simulink model "Observer_design"  (R2022a)
settings: Solver=ode45  StartTime=0.0  StopTime=30  RelTol=1e-3
values from neighbouring files (symbols this model uses):
  A = [0 0 1 0 0 ... (first row only)    [DesignProjectP2.m]    (also in DesignProjectP3.m; DesignProject_OffsetP3.m; mpc_example_regulation.m = [ 	 0,       0,              1,  0, 0; 	 0,       0,        ; mpc_example_tracking.m = [ 	 0,       0,              1,  0, 0; 	 0,       0,        )
  A_11 = A_measured(:,1:2)    [DesignProjectP2.m]
  A_12 = A_measured(:,3:5)    [DesignProjectP2.m]
  A_21 = A_estimated(:,1:2)    [DesignProjectP2.m]
  A_22 = A_estimated(:,3:5)    [DesignProjectP2.m]
  absolute_encoder_counts_per_revolution = 4096    [ELEN90064_Project_Parameters.m]
  B = [0;0;0;0;1/La]    [DesignProjectP2.m]    (also in DesignProjectP3.m; DesignProject_OffsetP3.m; mpc_example_regulation.m = [0; 0; 0; 0; 1/La]; mpc_example_tracking.m = [0; 0; 0; 0; 1/La])
  B_1 = [Dp.b(1); Dp.b(2)]    [DesignProjectP2.m]
  B_2 = [Dp.b(3); Dp.b(4); Dp.b(5)]    [DesignProjectP2.m]
  C = [1 0 0 0 0 ... (first row only)    [DesignProjectP2.m]    (also in DesignProjectP3.m; DesignProject_OffsetP3.m; mpc_example_regulation.m; mpc_example_tracking.m)
  Dp = c2d(Gp, T, 'zoh')    [DesignProjectP2.m]    (also in DesignProject_OffsetP3.m; mpc_example_regulation.m; mpc_example_tracking.m)
  init = [theta_m_init; theta_l_init; thetadot_m_init; thetadot_l_init; Ia_init]    [ELEN90064_Project_Parameters.m]
  J_r = place(A_22', A_12', obsz)'    [DesignProjectP2.m]
  L = place(A', C', observer_poles)'    [DesignProjectP2.m]    (also in DesignProjectP3.m; DesignProject_OffsetP3.m = L_t'; phase2_emc.m = place(A',C',desired_obsv_poles)')
  T = 1/50    (= 0.02)    [DesignProjectP2.m]    (also in DesignProject_OffsetP3.m; mpc_example_regulation.m; mpc_example_tracking.m)
  theta_l_init = deg2rad(0)    [ELEN90064_Project_Parameters.m]    (also in mpc_example_regulation.m; mpc_example_tracking.m)
  vision_fps = 50    [ELEN90064_Project_Parameters.m]
settings Model: Creator=Admin  LastModifiedBy=Admin

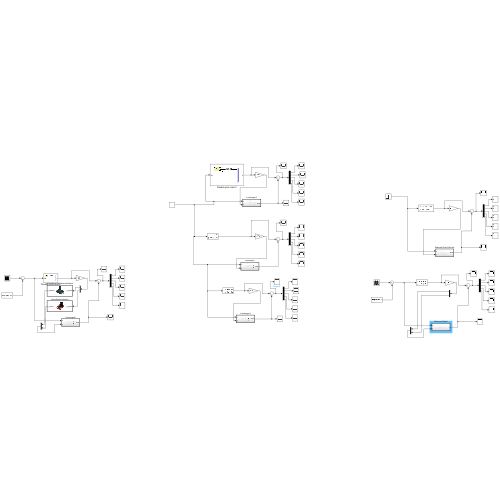
[thumbnail: Simulink's stored preview of the top-level diagram]
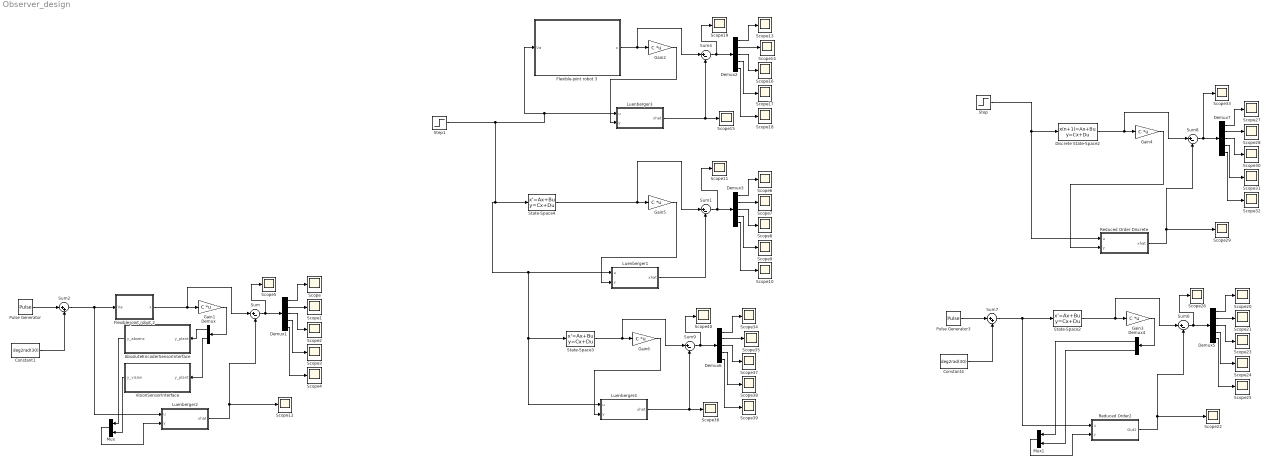
== system Observer_design ==
  AbsoluteEncoderSensorInterface : Subsystem  TreatAsAtomicUnit=on
      mask Display: image('$imagefile'); % Use "Edit Image" on toolstrip to change.
  Constant1 : Constant  Value=deg2rad(30)
  Constant4 : Constant  Value=deg2rad(30)
  Demux : Demux  Outputs=2
  Demux{1..3,5..7} (6 alike) : Demux  Outputs=5
  Demux4 : Demux  Outputs=2
  Discrete State-Space2 : DiscreteStateSpace  A=Dp.a  B=Dp.b  C=Dp.c  D=Dp.d  SampleTime=T
  Flexible-joint robot 2 : Subsystem
      mask Display: image('$imagefile'); % Use "Edit Image" on toolstrip to change.
  Flexible-joint robot 3 : Subsystem
      mask Display: image('$imagefile'); % Use "Edit Image" on toolstrip to change.
  Gain{1..6} (6 alike) : Gain  Gain=C  Multiplication=Matrix(K*u)
  Luenberger1 : Subsystem  TreatAsAtomicUnit=on
  Luenberger2 : Subsystem  TreatAsAtomicUnit=on
  Luenberger3 : Subsystem  TreatAsAtomicUnit=on
  Luenberger4 : Subsystem  TreatAsAtomicUnit=on
  Mux : Mux  Inputs=2
  Mux1 : Mux  Inputs=2
  Pulse Generator : DiscretePulseGenerator  PulseType=Time based  Amplitude=deg2rad(30)  Period=10  PulseWidth=50
  Pulse Generator3 : DiscretePulseGenerator  PulseType=Time based  Amplitude=deg2rad(30)  Period=10  PulseWidth=50
  Reduced Order Discrete : Subsystem  TreatAsAtomicUnit=on
  Reduced Order2 : Subsystem  TreatAsAtomicUnit=on
  Scope{,1..40} (41 alike) : Scope
  State-Space2 : StateSpace  A=A  B=B  C=eye(5)  D=zeros(5,1)  InitialCondition=0
  State-Space3 : StateSpace  A=A  B=B  C=eye(5)  D=zeros(5,1)  InitialCondition=0
  State-Space4 : StateSpace  A=A  B=B  C=eye(5)  D=zeros(5,1)  InitialCondition=0
  Step : Step  Time=deg2rad(60)  SampleTime=0
  Step1 : Step  Time=deg2rad(60)  SampleTime=0
  Sum{,1,4,6,8..9} (6 alike) : Sum  Inputs=|+-
  Sum2 : Sum  Inputs=|++
  Sum7 : Sum  Inputs=|++
  VisionSensorInterface : Subsystem  TreatAsAtomicUnit=on
      mask Display: image('$imagefile'); % Use "Edit Image" on toolstrip to change.
  wires:
  Constant1/1 -> Sum2/2
  Pulse Generator/1 -> Sum2/1
  Flexible-joint robot 2/1(x) -> Gain1/1, Sum/1
  Luenberger2/1(xhat) -> Sum/2, Scope12/1
  Sum/1 -> Scope5/1, Demux1/1
  Demux1/1 -> Scope/1
  Demux1/2 -> Scope1/1
  Demux1/3 -> Scope2/1
  Demux1/4 -> Scope3/1
  Demux1/5 -> Scope4/1
  Gain1/1 -> Demux/1
  Sum2/1 -> Flexible-joint robot 2/1(Va), Luenberger2/1(u)
  Demux3/5 -> Scope10/1
  Demux3/1 -> Scope6/1
  Gain5/1 -> Luenberger1/2(y)
  Demux3/3 -> Scope8/1
  Demux3/4 -> Scope9/1
  Sum1/1 -> Scope11/1, Demux3/1
  Luenberger1/1(xhat) -> Sum1/2
  Demux3/2 -> Scope7/1
  State-Space4/1 -> Gain5/1, Sum1/1
  Flexible-joint robot 3/1(x) -> Gain2/1, Sum4/1
  Gain2/1 -> Luenberger3/2(y)
  Demux2/5 -> Scope18/1
  Demux2/4 -> Scope17/1
  Demux2/2 -> Scope14/1
  Sum4/1 -> Scope19/1, Demux2/1
  Demux2/3 -> Scope16/1
  Demux2/1 -> Scope13/1
  Luenberger3/1(xhat) -> Scope15/1, Sum4/2
  AbsoluteEncoderSensorInterface/1(y_absenc) -> Mux/1
  Demux/1 -> AbsoluteEncoderSensorInterface/1(y_plant)
  Mux/1 -> Luenberger2/2(y)
  Mux1/1 -> Reduced Order2/2(y)
  Demux4/2 -> Mux1/2
  Demux4/1 -> Mux1/1
  Sum7/1 -> Reduced Order2/1(u), State-Space2/1
  Gain3/1 -> Demux4/1
  Demux5/5 -> Scope25/1
  Demux5/4 -> Scope24/1
  Demux5/3 -> Scope23/1
  Demux5/2 -> Scope21/1
  Demux5/1 -> Scope20/1
  Sum6/1 -> Demux5/1, Scope26/1
  Reduced Order2/1(Out1) -> Scope22/1, Sum6/2
  State-Space2/1 -> Sum6/1, Gain3/1
  Pulse Generator3/1 -> Sum7/1
  Constant4/1 -> Sum7/2
  Demux/2 -> VisionSensorInterface/1(y_plant)
  VisionSensorInterface/1(y_vision) -> Mux/2
  Discrete State-Space2/1 -> Gain4/1, Sum8/1
  Reduced Order Discrete/1(xhat) -> Sum8/2, Scope29/1
  Sum8/1 -> Scope33/1, Demux7/1
  Demux7/1 -> Scope27/1
  Demux7/2 -> Scope28/1
  Demux7/3 -> Scope30/1
  Demux7/4 -> Scope31/1
  Demux7/5 -> Scope32/1
  Step/1 -> Discrete State-Space2/1, Reduced Order Discrete/1(u)
  Gain4/1 -> Reduced Order Discrete/2(y)
  Luenberger4/1(xhat) -> Sum9/2, Scope36/1
  Demux6/1 -> Scope34/1
  Demux6/3 -> Scope37/1
  Sum9/1 -> Demux6/1, Scope40/1
  Demux6/2 -> Scope35/1
  Demux6/4 -> Scope38/1
  Demux6/5 -> Scope39/1
  Step1/1 -> State-Space4/1, State-Space3/1, Luenberger4/1(u), Luenberger1/1(u), Flexible-joint robot 3/1(Va), Luenberger3/1(u)
  Gain6/1 -> Luenberger4/2(y)
  State-Space3/1 -> Sum9/1, Gain6/1

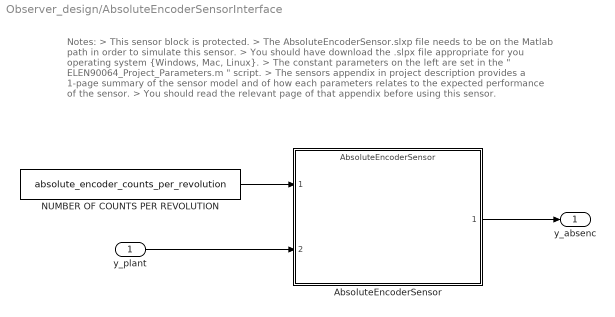
== system Observer_design/AbsoluteEncoderSensorInterface ==
  note: Notes:
      | > This sensor block is protected.
      | > The AbsoluteEncoderSensor.slxp file needs to be on the Matlab path in order to simulate this sensor.
      | > You should have download the .slpx file appropriate for you operating system {Windows, Mac, Linux}.
      | > The constant parameters on the left are set in the " ELEN90064_Project_Parameters.m " script.
      | > The sensors appendix in project description provides a 1-page summary of the sensor model and of how each parameters relates to the expected performance of the sensor.
      | > You should read the relevant page of that appendix before using this sensor.
  y_plant : Inport
  AbsoluteEncoderSensor : ModelReference  ModelNameDialog=AbsoluteEncoderSensor.slxp  ModelReferenceVersion=1.16  CopyOfModelProtected=on
  NUMBER OF COUNTS PER REVOLUTION : Constant  Value=absolute_encoder_counts_per_revolution
  y_absenc : Outport
  wires:
  NUMBER OF COUNTS PER REVOLUTION/1 -> AbsoluteEncoderSensor/1
  y_plant/1 -> AbsoluteEncoderSensor/2
  AbsoluteEncoderSensor/1 -> y_absenc/1

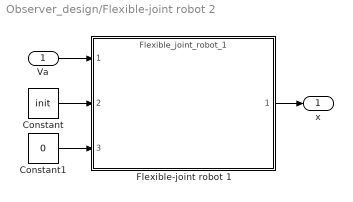
== system Observer_design/Flexible-joint robot 2 ==
  Va : Inport
  Constant : Constant  Value=init
  Constant1 : Constant  Value=0
  Flexible-joint robot 1 : ModelReference  ModelNameDialog=Flexible_joint_robot_1  ModelReferenceVersion=1.65  CopyOfModelProtected=on
  x : Outport
  wires:
  Va/1 -> Flexible-joint robot 1/1
  Flexible-joint robot 1/1 -> x/1
  Constant1/1 -> Flexible-joint robot 1/3
  Constant/1 -> Flexible-joint robot 1/2

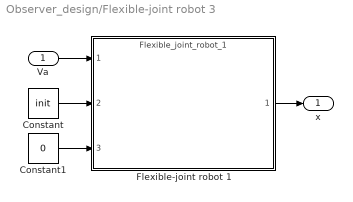
== system Observer_design/Flexible-joint robot 3 ==
  Va : Inport
  Constant : Constant  Value=init
  Constant1 : Constant  Value=0
  Flexible-joint robot 1 : ModelReference  ModelNameDialog=Flexible_joint_robot_1  ModelReferenceVersion=1.65  CopyOfModelProtected=on
  x : Outport
  wires:
  Va/1 -> Flexible-joint robot 1/1
  Flexible-joint robot 1/1 -> x/1
  Constant1/1 -> Flexible-joint robot 1/3
  Constant/1 -> Flexible-joint robot 1/2

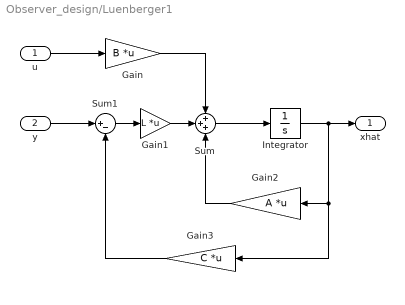
== system Observer_design/Luenberger1 ==
  u : Inport
  y : Inport  Port=2
  Gain : Gain  Gain=B  Multiplication=Matrix(K*u) (u vector)
  Gain1 : Gain  Gain=L  Multiplication=Matrix(K*u) (u vector)
  Gain2 : Gain  Gain=A  Multiplication=Matrix(K*u) (u vector)
  Gain3 : Gain  Gain=C  Multiplication=Matrix(K*u) (u vector)
  Integrator : Integrator
  Sum : Sum  Inputs=+++
  Sum1 : Sum  Inputs=|+-
  xhat : Outport
  wires:
  u/1 -> Gain/1
  Gain/1 -> Sum/1
  y/1 -> Sum1/1
  Sum1/1 -> Gain1/1
  Gain1/1 -> Sum/2
  Sum/1 -> Integrator/1
  Integrator/1 -> Gain3/1, Gain2/1, xhat/1
  Gain2/1 -> Sum/3
  Gain3/1 -> Sum1/2

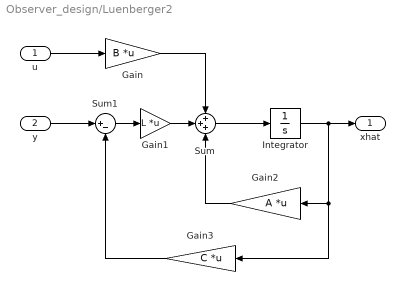
== system Observer_design/Luenberger2 ==
  u : Inport
  y : Inport  Port=2
  Gain : Gain  Gain=B  Multiplication=Matrix(K*u) (u vector)
  Gain1 : Gain  Gain=L  Multiplication=Matrix(K*u) (u vector)
  Gain2 : Gain  Gain=A  Multiplication=Matrix(K*u) (u vector)
  Gain3 : Gain  Gain=C  Multiplication=Matrix(K*u) (u vector)
  Integrator : Integrator
  Sum : Sum  Inputs=+++
  Sum1 : Sum  Inputs=|+-
  xhat : Outport
  wires:
  u/1 -> Gain/1
  Gain/1 -> Sum/1
  y/1 -> Sum1/1
  Sum1/1 -> Gain1/1
  Gain1/1 -> Sum/2
  Sum/1 -> Integrator/1
  Integrator/1 -> Gain3/1, Gain2/1, xhat/1
  Gain2/1 -> Sum/3
  Gain3/1 -> Sum1/2

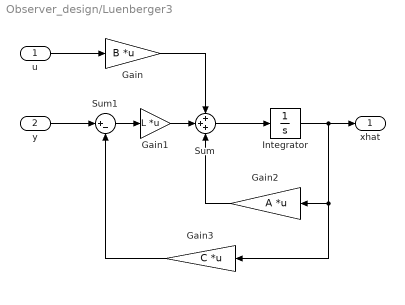
== system Observer_design/Luenberger3 ==
  u : Inport
  y : Inport  Port=2
  Gain : Gain  Gain=B  Multiplication=Matrix(K*u) (u vector)
  Gain1 : Gain  Gain=L  Multiplication=Matrix(K*u) (u vector)
  Gain2 : Gain  Gain=A  Multiplication=Matrix(K*u) (u vector)
  Gain3 : Gain  Gain=C  Multiplication=Matrix(K*u) (u vector)
  Integrator : Integrator
  Sum : Sum  Inputs=+++
  Sum1 : Sum  Inputs=|+-
  xhat : Outport
  wires:
  Gain3/1 -> Sum1/2
  Gain2/1 -> Sum/3
  Integrator/1 -> xhat/1, Gain2/1, Gain3/1
  Sum/1 -> Integrator/1
  Gain1/1 -> Sum/2
  Sum1/1 -> Gain1/1
  y/1 -> Sum1/1
  Gain/1 -> Sum/1
  u/1 -> Gain/1

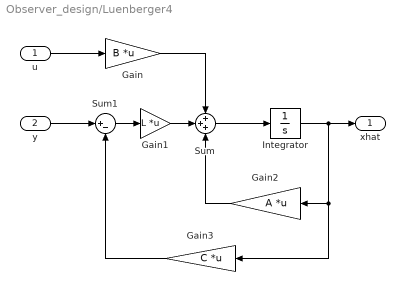
== system Observer_design/Luenberger4 ==
  u : Inport
  y : Inport  Port=2
  Gain : Gain  Gain=B  Multiplication=Matrix(K*u) (u vector)
  Gain1 : Gain  Gain=L  Multiplication=Matrix(K*u) (u vector)
  Gain2 : Gain  Gain=A  Multiplication=Matrix(K*u) (u vector)
  Gain3 : Gain  Gain=C  Multiplication=Matrix(K*u) (u vector)
  Integrator : Integrator
  Sum : Sum  Inputs=+++
  Sum1 : Sum  Inputs=|+-
  xhat : Outport
  wires:
  u/1 -> Gain/1
  Gain/1 -> Sum/1
  y/1 -> Sum1/1
  Sum1/1 -> Gain1/1
  Gain1/1 -> Sum/2
  Sum/1 -> Integrator/1
  Integrator/1 -> Gain3/1, Gain2/1, xhat/1
  Gain2/1 -> Sum/3
  Gain3/1 -> Sum1/2

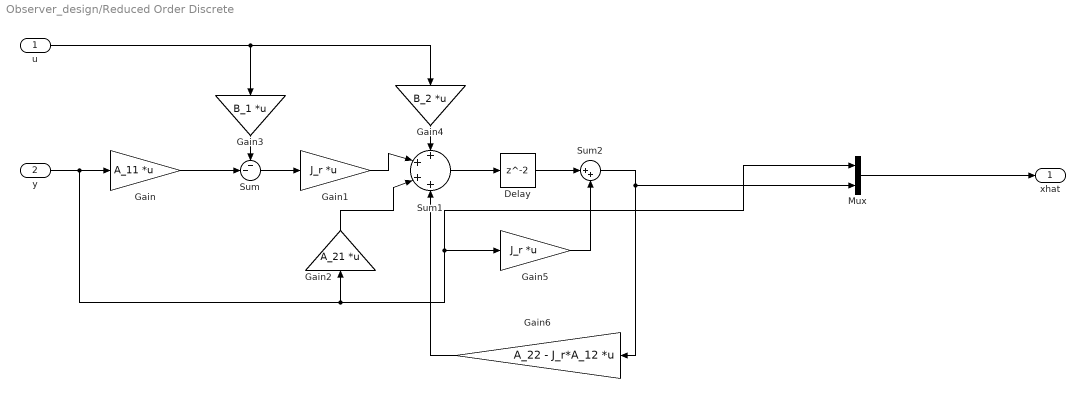
== system Observer_design/Reduced Order Discrete ==
  u : Inport
  y : Inport  Port=2
  Delay : Delay
  Gain : Gain  Gain=A_11  Multiplication=Matrix(K*u) (u vector)
  Gain1 : Gain  Gain=J_r  Multiplication=Matrix(K*u) (u vector)
  Gain2 : Gain  Gain=A_21  Multiplication=Matrix(K*u) (u vector)
  Gain3 : Gain  Gain=B_1  Multiplication=Matrix(K*u) (u vector)
  Gain4 : Gain  Gain=B_2  Multiplication=Matrix(K*u) (u vector)
  Gain5 : Gain  Gain=J_r  Multiplication=Matrix(K*u) (u vector)
  Gain6 : Gain  Gain=A_22 - J_r*A_12  Multiplication=Matrix(K*u) (u vector)
  Mux : Mux  Inputs=2
  Sum : Sum  Inputs=--|
  Sum1 : Sum  Inputs=++++
  Sum2 : Sum  Inputs=|++
  xhat : Outport
  wires:
  Mux/1 -> xhat/1
  Sum2/1 -> Mux/2, Gain6/1
  Gain6/1 -> Sum1/4
  Delay/1 -> Sum2/1
  Gain5/1 -> Sum2/2
  Sum1/1 -> Delay/1
  Gain4/1 -> Sum1/1
  Gain3/1 -> Sum/1
  Gain2/1 -> Sum1/3
  Gain1/1 -> Sum1/2
  Sum/1 -> Gain1/1
  Gain/1 -> Sum/2
  y/1 -> Gain/1, Mux/1, Gain5/1, Gain2/1
  u/1 -> Gain3/1, Gain4/1

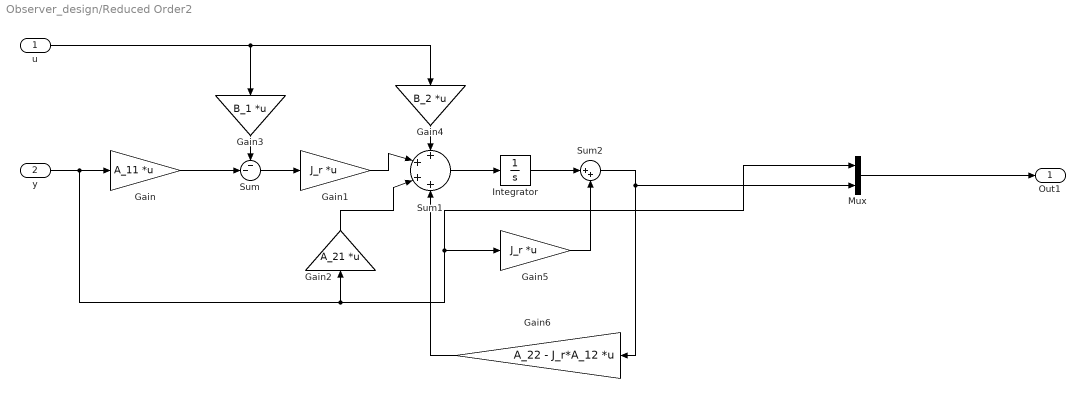
== system Observer_design/Reduced Order2 ==
  u : Inport
  y : Inport  Port=2
  Gain : Gain  Gain=A_11  Multiplication=Matrix(K*u) (u vector)
  Gain1 : Gain  Gain=J_r  Multiplication=Matrix(K*u) (u vector)
  Gain2 : Gain  Gain=A_21  Multiplication=Matrix(K*u) (u vector)
  Gain3 : Gain  Gain=B_1  Multiplication=Matrix(K*u) (u vector)
  Gain4 : Gain  Gain=B_2  Multiplication=Matrix(K*u) (u vector)
  Gain5 : Gain  Gain=J_r  Multiplication=Matrix(K*u) (u vector)
  Gain6 : Gain  Gain=A_22 - J_r*A_12  Multiplication=Matrix(K*u) (u vector)
  Integrator : Integrator
  Mux : Mux  Inputs=2
  Sum : Sum  Inputs=--|
  Sum1 : Sum  Inputs=++++
  Sum2 : Sum  Inputs=|++
  Out1 : Outport
  wires:
  u/1 -> Gain4/1, Gain3/1
  y/1 -> Gain2/1, Gain5/1, Mux/1, Gain/1
  Gain/1 -> Sum/2
  Sum/1 -> Gain1/1
  Gain1/1 -> Sum1/2
  Gain2/1 -> Sum1/3
  Gain3/1 -> Sum/1
  Gain4/1 -> Sum1/1
  Sum1/1 -> Integrator/1
  Gain5/1 -> Sum2/2
  Integrator/1 -> Sum2/1
  Gain6/1 -> Sum1/4
  Sum2/1 -> Gain6/1, Mux/2
  Mux/1 -> Out1/1

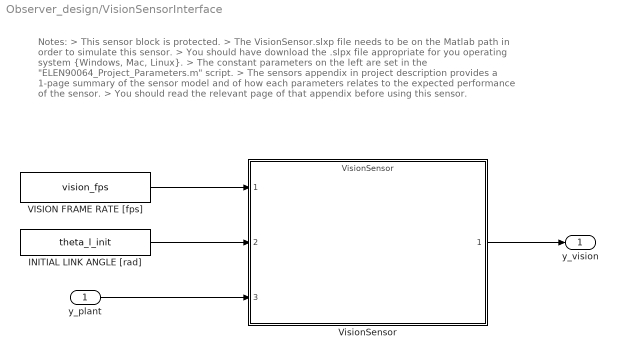
== system Observer_design/VisionSensorInterface ==
  note: Notes:
      | > This sensor block is protected.
      | > The VisionSensor.slxp file needs to be on the Matlab path in order to simulate this sensor.
      | > You should have download the .slpx file appropriate for you operating system {Windows, Mac, Linux}.
      | > The constant parameters on the left are set in the "ELEN90064_Project_Parameters.m" script.
      | > The sensors appendix in project description provides a 1-page summary of the sensor model and of how each parameters relates to the expected performance of the sensor.
      | > You should read the relevant page of that appendix before using this sensor.
  y_plant : Inport
  INITIAL LINK ANGLE [rad] : Constant  Value=theta_l_init
  VISION FRAME RATE [fps] : Constant  Value=vision_fps
  VisionSensor : ModelReference  ModelNameDialog=VisionSensor.slxp  ModelReferenceVersion=1.19  CopyOfModelProtected=on
  y_vision : Outport
  wires:
  VISION FRAME RATE [fps]/1 -> VisionSensor/1
  INITIAL LINK ANGLE [rad]/1 -> VisionSensor/2
  y_plant/1 -> VisionSensor/3
  VisionSensor/1 -> y_vision/1
